simulink model "mnist_cnn_adam"  (R2017b)
settings: Solver=FixedStepDiscrete  StartTime=0.0  StopTime=2  FixedStep=1  RelTol=1e-3
model workspace (MATLAB code in the model file):
  | filtersize1 = 5;
  | filtersize2 = 5;
  | features1 = 16;
  | features2 = 16;
  | densesize = 64;
  | classes = 10;
  | batchsize = 64;
libraries: ad_blocks x27
settings Model: PauseTimes=2  SnapshotBufferSize=2  SnapshotInterval=1  Creator=percro2  LastModifiedBy=eruffaldi
settings RTWCC: GenerateReport=on  LaunchReport=on
settings CodeAppCC: StateflowObjectComments=on  MATLABSourceComments=on

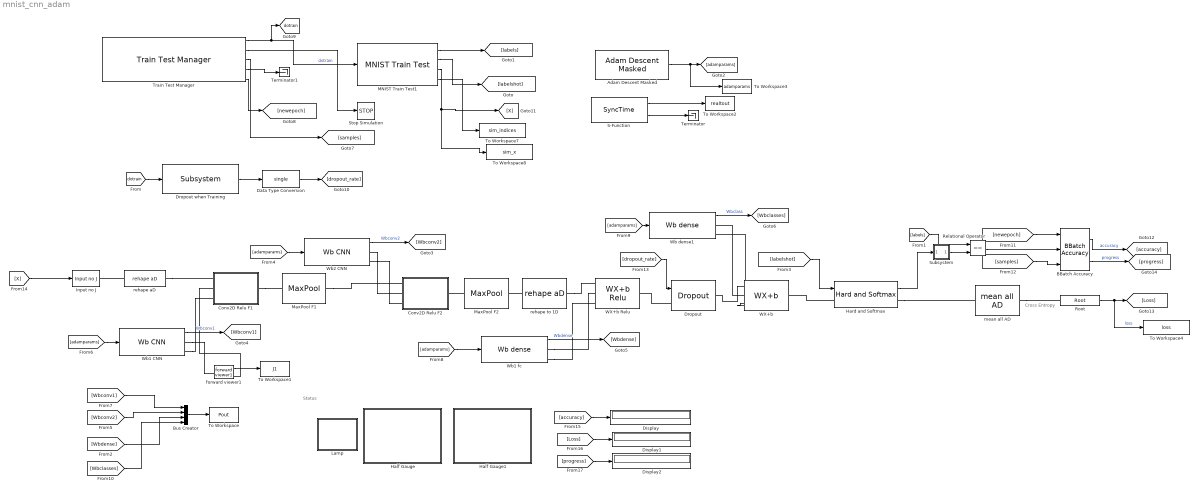
== system mnist_cnn_adam ==
  note: Cross Entropy
  note: Status
  Adam Descent Masked : ad_blocks/Adam Descent Masked  learningrate=1e-4  beta1=0.9  beta2=0.9999  epsilon=1e-8  adam=on
  BBatch Accuracy : ad_blocks/BBatch Accuracy
  Bus Creator : BusCreator  Inputs=4
  Conv2D Relu F1 : Subsystem
  Conv2D Relu F2 : Subsystem
  Data Type Conversion : DataTypeConversion  OutDataTypeStr=single
  Display : Display
  Display1 : Display
  Display2 : Display
  Dropout : ad_blocks/Dropout
  Dropout when Training : ad_blocks/Subsystem  dropout_rate=0.8
  Half Gauge : Subsystem  DialogController=hmiCreateDDGDialog  IsWebBlock=on  mask(MWDashboardBlock){webBlockId=3ccc98f6-79d6-4568-b009-3c502e494738, webBlockType=semicirculargauge, ShowInLibBrowser=on, ShowInitialText=on, HMISrcModelName=mnist_cnn_adam}
      mask prompts: webBlockId "WebBlock Id"; webBlockType "WebBlock Type"; HMISrcModelName "Source Model"
      mask help: SimulinkHMI:dialogs:SemicircularGaugeDialogDesc
      mask Help: helpview([docroot '/mapfiles/simulink.map'], 'hmi_half_gauge')
      mask Display:
      | if strcmp(get_param(bdroot(gcb),'BlockDiagramType'), 'library')
      |     image([(matlabroot) '/toolbox/simulink/hmi/icons/SemicircularGauge.png']);
      | end
  Half Gauge1 : Subsystem  DialogController=hmiCreateDDGDialog  IsWebBlock=on  mask(MWDashboardBlock){webBlockId=9a81c562-48ac-4438-82f8-4bec04368701, webBlockType=semicirculargauge, ShowInLibBrowser=on, ShowInitialText=on, HMISrcModelName=mnist_cnn_adam}
      mask prompts: webBlockId "WebBlock Id"; webBlockType "WebBlock Type"; HMISrcModelName "Source Model"
      mask help: SimulinkHMI:dialogs:SemicircularGaugeDialogDesc
      mask Help: helpview([docroot '/mapfiles/simulink.map'], 'hmi_half_gauge')
      mask Display:
      | if strcmp(get_param(bdroot(gcb),'BlockDiagramType'), 'library')
      |     image([(matlabroot) '/toolbox/simulink/hmi/icons/SemicircularGauge.png']);
      | end
  Hard and Softmax : ad_blocks/Hard and Softmax
  Input no J : ad_blocks/Input no J  SystemSampleTime=-1
  Lamp : Subsystem  DialogController=hmiCreateDDGDialog  IsWebBlock=on  mask(MWDashboardBlock){webBlockId=47d178a8-8845-4c3e-9db8-10541501d251, webBlockType=lamp, ShowInLibBrowser=on, ShowInitialText=on, HMISrcModelName=mnist_cnn_adam}
      mask prompts: webBlockType "WebBlock Type"; HMISrcModelName "Source Model"
      mask help: SimulinkHMI:dialogs:LampDialogDesc
      mask Help: helpview([docroot '/mapfiles/simulink.map'], 'hmi_lamp')
      mask Display:
      | if strcmp(get_param(bdroot(gcb),'BlockDiagramType'), 'library')
      |     image([(matlabroot) '/toolbox/simulink/hmi/icons/Lamp.png']);
      | end
  MNIST Train Test1 : ad_blocks/MNIST Train Test  mask{BatchSize=batchsize}
  MaxPool F1 : ad_blocks/MaxPool  stride=[1,2,2,1]  ksize=[1,2,2,1]  padding=-1
  MaxPool F2 : ad_blocks/MaxPool  stride=[1,2,2,1]  ksize=[1,2,2,1]  padding=-1
  Relational Operator : RelationalOperator  Operator===  OutDataTypeStr=boolean  RndMeth=Simplest
  Root : ad_blocks/Root  Description=Top level AD block: gets the incoming value, pushes the scalar 1 gradient  SystemSampleTime=-1
  S-Function : S-Function  Priority=1024  FunctionName=SyncTime  Parameters=dt  SFunctionDeploymentMode=off  EnableBusSupport=off  mask{dt=0}
      mask prompts: dt "Period (s) or 0 for sleepless"
      mask Display:
      | port_label('output',1,'Unix Epoch s');
      | port_label('output',2,'Slept s');
  Stop Simulation : Stop
  Subsystem : Subsystem
  Terminator : Terminator
  Terminator1 : Terminator
  To Workspace : ToWorkspace  VariableName=Pout  SaveFormat=Timeseries  SampleTime=-1
      settings: MaxDataPoints=3
  To Workspace1 : ToWorkspace  VariableName=J1  SaveFormat=Timeseries  SampleTime=-1
      settings: MaxDataPoints=3
  To Workspace2 : ToWorkspace  VariableName=realtout  SaveFormat=Timeseries  SampleTime=1
  To Workspace3 : ToWorkspace  VariableName=adamparams  SaveFormat=Timeseries  SampleTime=1
      settings: MaxDataPoints=2
  To Workspace4 : ToWorkspace  VariableName=loss  SaveFormat=Timeseries  SampleTime=-1
      settings: MaxDataPoints=3
  To Workspace7 : ToWorkspace  VariableName=sim_indices  SaveFormat=Timeseries  SampleTime=-1
      settings: MaxDataPoints=1
  To Workspace8 : ToWorkspace  VariableName=sim_x  SaveFormat=Timeseries  SampleTime=-1
      settings: MaxDataPoints=1
  Train Test Manager : ad_blocks/Train Test Manager  testsize=10000  trainsize=60000  skiptrain=0  epochs=2  batchsize=batchsize  SimulateUsing=Code generation
  "WX+b " : ad_blocks/WX+b 
  WX+b Relu : ad_blocks/WX+b Relu
  Wb dense1 : ad_blocks/Wb dense  wshape=[densesize,classes]
  Wb1 CNN : ad_blocks/Wb CNN  K=filtersize1  Fi=1  Fo=features1
  Wb1 fc : ad_blocks/Wb dense  wshape=[7*7*features2,densesize]
  Wb2 CNN : ad_blocks/Wb CNN  K=filtersize2  Fi=features1  Fo=features2
  forward viewer1 : ad_blocks/forward viewer1  SystemSampleTime=-1
  mean all AD : ad_blocks/mean all AD
  rehape aD : ad_blocks/rehape aD  shape=[-1,28,28]
  rehape to 1D : ad_blocks/rehape aD  shape=[-1,-1]
  tag scope: dotrain=global
  wires:
  [labels] -> Relational Operator/1
  S-Function/1 -> To Workspace2/1
  S-Function/2 -> Terminator/1
  Bus Creator/1 -> To Workspace/1
  Wb2 CNN/1 -> [Wbconv2]  "Wbconv2"
  [adamparams] -> Wb2 CNN/1
  [Wbconv2] -> Bus Creator/2
  [adamparams] -> Wb1 CNN/1
  [Wbconv1] -> Bus Creator/1
  Wb1 CNN/1 -> [Wbconv1]  "Wbconv1"
  Wb1 fc/1 -> [Wbdense]  "Wbdense"
  [adamparams] -> Wb1 fc/1
  Wb dense1/1 -> [Wbclasses]  "Wbclass"
  [adamparams] -> Wb dense1/1
  [Wbdense] -> Bus Creator/3
  [Wbclasses] -> Bus Creator/4
  Train Test Manager/5 -> [newepoch]
  Train Test Manager/1 -> [dotrain], MNIST Train Test1/1  "dotrain"
  Train Test Manager/3 -> [samples]
  MNIST Train Test1/1 -> [labels]
  MNIST Train Test1/4 -> To Workspace7/1
  MNIST Train Test1/3 -> [X], To Workspace8/1
  MNIST Train Test1/2 -> [labelshot]
  Train Test Manager/2 -> Stop Simulation/1
  [newepoch] -> BBatch Accuracy/1
  Relational Operator/1 -> BBatch Accuracy/2
  [samples] -> BBatch Accuracy/3
  Dropout when Training/1 -> Data Type Conversion/1
  [dropout_rate] -> Dropout/1
  Train Test Manager/4 -> Terminator1/1
  [dotrain] -> Dropout when Training/1
  Data Type Conversion/1 -> [dropout_rate]
  [X] -> Input no J/1
  BBatch Accuracy/1 -> [accuracy]  "accuracy"
  Root/1 -> To Workspace4/1, [Loss]  "loss"
  [accuracy] -> Display/1
  [Loss] -> Display1/1
  [labelshot] -> Hard and Softmax/1
  Hard and Softmax/1 -> Subsystem/1(In1)
  Adam Descent Masked/1 -> To Workspace3/1, [adamparams]
  Subsystem/1(Out1) -> Relational Operator/2
  forward viewer1/1 -> To Workspace1/1
  BBatch Accuracy/2 -> [progress]  "progress"
  [progress] -> Display2/1
  connections:
  rehape aD/LConn1 -- Input no J/RConn1
  mean all AD/RConn1 -- Root/LConn1
  MaxPool F2/LConn1 -- Conv2D Relu F2/RConn1
  rehape to 1D/LConn1 -- MaxPool F2/RConn1
  Dropout/LConn1 -- WX+b Relu/RConn1
  "WX+b "/LConn1 -- Dropout/RConn1
  "WX+b "/LConn2 -- Wb dense1/RConn1
  "WX+b "/LConn3 -- Wb dense1/RConn2
  Wb1 CNN/RConn2 -- Conv2D Relu F1/LConn3
  rehape to 1D/RConn1 -- WX+b Relu/LConn1
  Wb2 CNN/RConn1 -- Conv2D Relu F2/LConn2
  Wb2 CNN/RConn2 -- Conv2D Relu F2/LConn3
  Wb1 fc/RConn1 -- WX+b Relu/LConn2
  Wb1 fc/RConn2 -- WX+b Relu/LConn3
  Hard and Softmax/LConn1 -- "WX+b "/RConn1
  Hard and Softmax/RConn1 -- mean all AD/LConn1
  MaxPool F1/RConn1 -- Conv2D Relu F2/LConn1
  Conv2D Relu F1/RConn1 -- MaxPool F1/LConn1
  rehape aD/RConn1 -- Conv2D Relu F1/LConn1
  Wb1 CNN/RConn1 -- forward viewer1/LConn1
  forward viewer1/RConn1 -- Conv2D Relu F1/LConn2

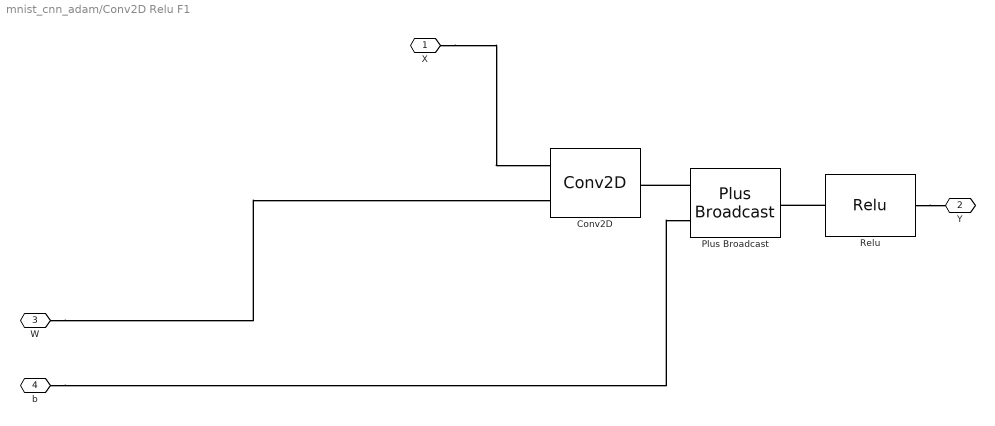
== system mnist_cnn_adam/Conv2D Relu F1 ==
  Conv2D : ad_blocks/Conv2D  stride=[1,1,1,1]  padding=-1
  Plus Broadcast : ad_blocks/Plus Broadcast
  Relu : ad_blocks/Relu
  X : PMIOPort  Port=1  Side=Left
  Y : PMIOPort  Port=2  Side=Right
  W : PMIOPort  Port=3  Side=Left
  b : PMIOPort  Port=4  Side=Left
  connections:
  Relu/LConn1 -- Plus Broadcast/RConn1
  Plus Broadcast/LConn1 -- Conv2D/RConn1
  Relu/RConn1 -- Y/RConn1
  b/RConn1 -- Plus Broadcast/LConn2
  X/RConn1 -- Conv2D/LConn1
  W/RConn1 -- Conv2D/LConn2

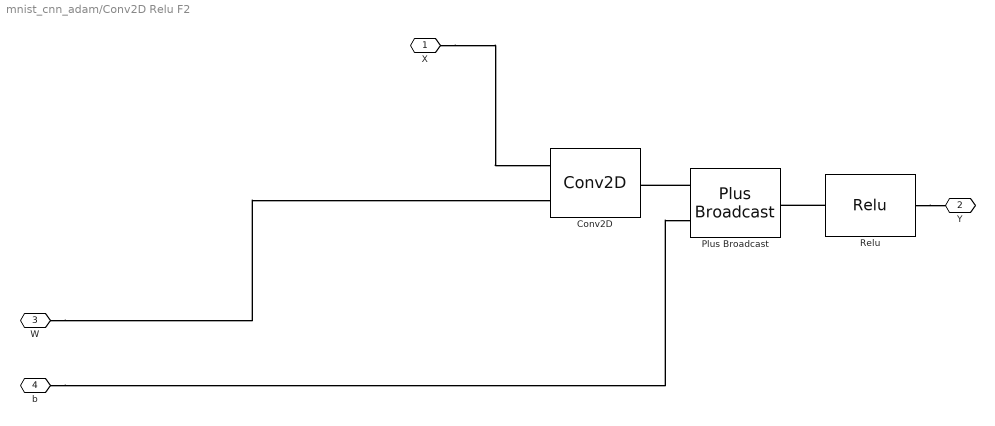
== system mnist_cnn_adam/Conv2D Relu F2 ==
  Conv2D : ad_blocks/Conv2D  stride=[1,1,1,1]  padding=-1
  Plus Broadcast : ad_blocks/Plus Broadcast
  Relu : ad_blocks/Relu
  X : PMIOPort  Port=1  Side=Left
  Y : PMIOPort  Port=2  Side=Right
  W : PMIOPort  Port=3  Side=Left
  b : PMIOPort  Port=4  Side=Left
  connections:
  W/RConn1 -- Conv2D/LConn2
  X/RConn1 -- Conv2D/LConn1
  b/RConn1 -- Plus Broadcast/LConn2
  Relu/RConn1 -- Y/RConn1
  Plus Broadcast/LConn1 -- Conv2D/RConn1
  Relu/LConn1 -- Plus Broadcast/RConn1

== system mnist_cnn_adam/Half Gauge ==

== system mnist_cnn_adam/Half Gauge1 ==

== system mnist_cnn_adam/Lamp ==

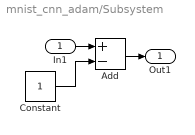
== system mnist_cnn_adam/Subsystem ==
  In1 : Inport
  Add : Sum  Inputs=+-
  Constant : Constant  OutDataTypeStr=Inherit: Inherit via back propagation
  Out1 : Outport
  wires:
  In1/1 -> Add/1
  Add/1 -> Out1/1
  Constant/1 -> Add/2
